simulink model "Assignment_2_RateAdaptive_UART"  (R2020a)
settings: Solver=FixedStepAuto  StartTime=0.0  StopTime=10.0  FixedStep=1e-3  RelTol=1e-3  EnableMultiTasking=on
undefined symbols (not defined in the file): A0, A1, D0, D1, D10, D11, D12, D13, D2, D3, D4, D5, D6, D7, D8, D9, PTA0, PTA1, PTA2, PTB2, PTB23, PTB3, PTB9, PTC16, PTC17, PTC2, PTC3, PTC4, PTD0, PTD1, PTD2, PTD3
libraries: frdmk64flib x22, etargetslib x5, dspstat3 x1, simulink x1
settings Model: ExtModeTrigDuration=5  Creator=School  LastModifiedBy=riley
settings OptimizationCC: EnhancedBackFolding=on  PassReuseOutputArgsAs=Individual arguments  ZeroExternalMemoryAtStartup=off  ZeroInternalMemoryAtStartup=off  MaxStackSize=64  OptimizeBlockOrder=speed  DifferentSizesBufferReuse=on  OptimizationCustomize=off  EfficientTunableParamExpr=on
settings DebuggingCC: ParameterTunabilityLossMsg=error
settings HardwareCC: ProdBitPerPointer=32  ProdBitPerSizeT=32  ProdBitPerPtrDiffT=32  ProdLargestAtomicInteger=Long  ProdLargestAtomicFloat=Double  ProdWordSize=32  ProdHWDeviceType=ARM Compatible->ARM Cortex
settings SFSimCC: MATLABDynamicMemAlloc=off
settings RTWCC: SystemTargetFile=ert.tlc  HardwareBoard=NXP FRDM-K64F  TemplateMakefile=ert_default_tmf  Toolchain=GNU Tools for ARM Embedded Processors
settings CodeAppCC: ForceParamTrailComments=on  IgnoreCustomStorageClasses=off  OperatorAnnotations=on  SimulinkDataObjDesc=on  SFDataObjDesc=on  InsertBlockDesc=on

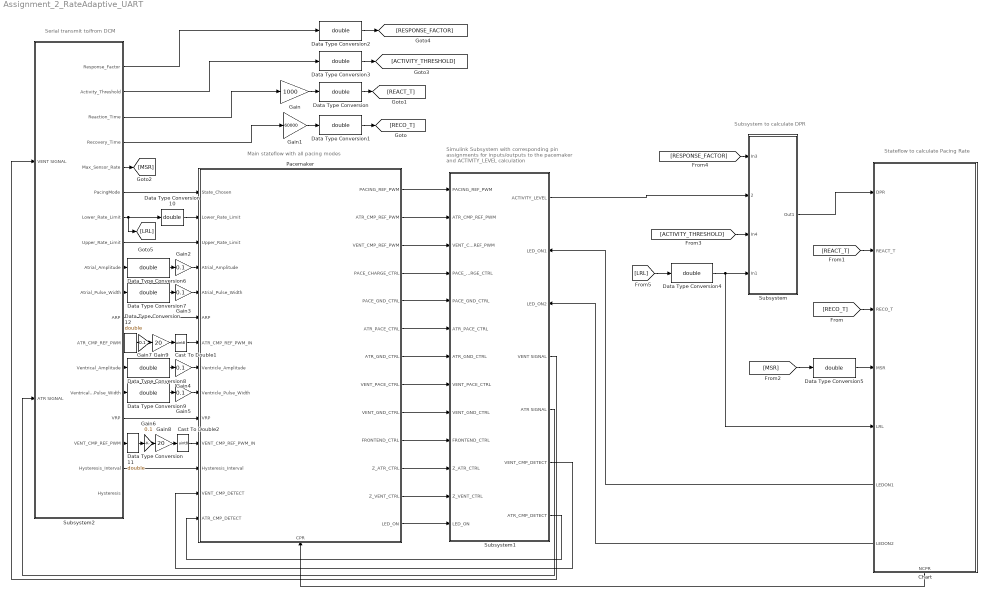
== system Assignment_2_RateAdaptive_UART ==
  note: Main stateflow with all pacing modes
  note: Serial transmit to/from DCM
  note: Stateflow to calculate Pacing Rate
  note: Subsystem to calculate DPR
  note: Simulink Subsystem with corresponding pin
      | assignments for inputs/outputs to the pacemaker
      | and ACTIVITY_LEVEL calculation
  Cast To Double1 : DataTypeConversion  OutDataTypeStr=uint8
  Cast To Double2 : DataTypeConversion  OutDataTypeStr=uint8
  Chart : Stateflow chart  TreatAsAtomicUnit=on
      settings: PortSchema="{\"entries\":[{\"content\":{\"sides\":[{\"content\":{\"connectorIds\":[\"In5\",\"In1\",\"In2\",\"In3\",\"In4\",\"Out2\",\"Out3\"]},\"type\":\"ConnectorPlacement.EquallySpacedRectSide\",\"uuid\":\"cb49ebd1-b2c7-4a1e-b062-18a1bf51e97f\"},{\"content\":{\"connectorIds\":[],\"side\":\"RIGHT\"},\"type\":\"ConnectorPlacement.EquallySpacedRectSide\",\"uuid\":\"35cf40a1-f02a-4965-9a15-2487395dd71b\"},{\"content\":{\"connectorIds\":[],\"side\":\"TOP\"},\"type\":\"ConnectorPlacement.EquallySpacedRectSide\",\"uuid\":\"8cf7664f-bebd-444c-a693-a1ee33fcaf3f\"},{\"content\":{\"connectorIds\":[\"Out1\"],\"side\":\"BOTTOM\"},\"type\":\"ConnectorPlacement.EquallySpacedRectSide\",\"uuid\":\"96b9c03b-a83e-462b-a12d-192e0bec7514\"}]},\"type\":\"ConnectorPlacement.EquallySpacedConnector\",\"uuid\":\"1030b27a-8fcd-482c-adda-aee1bfc69e16\"}],\"packageUris\":[\"http://schema.mathworks.com/mf0/Connector/19700101\"],\"version\":\"1.0\"}"
  Data Type Conversion{,1..12} (13 alike) : DataTypeConversion  OutDataTypeStr=double
  Gain : Gain  Gain=1000
  Gain1 : Gain  Gain=60000
  Gain{2..7} (6 alike) : Gain  Gain=0.1
  Gain8 : Gain  Gain=20
  Gain9 : Gain  Gain=20
  Pacemaker : Stateflow chart  TreatAsAtomicUnit=on
      settings: PortSchema="{\"entries\":[{\"content\":{\"sides\":[{\"content\":{\"connectorIds\":[\"In1\",\"In2\",\"In4\",\"In11\",\"In3\",\"In10\",\"In12\",\"In14\",\"In6\",\"In9\",\"In13\",\"In8\",\"In7\",\"In5\"]},\"type\":\"ConnectorPlacement.EquallySpacedRectSide\",\"uuid\":\"df877ca0-8245-4163-8fee-7182eab1d55d\"},{\"content\":{\"connectorIds\":[\"Out11\",\"Out12\",\"Out13\",\"Out2\",\"Out3\",\"Out1\",\"Out5\",\"Out7\",\"Out8\",\"Out10\",\"Out4\",\"Out9\",\"Out6\"],\"side\":\"RIGHT\"},\"type\":\"ConnectorPlacement.EquallySpacedRectSide\",\"uuid\":\"3a694184-6a85-4729-834f-a3ab7480664d\"},{\"content\":{\"connectorIds\":[],\"side\":\"TOP\"},\"type\":\"ConnectorPlacement.EquallySpacedRectSide\",\"uuid\":\"45b3d390-d3d3-4e22-8b52-b1590054c23a\"},{\"content\":{\"connectorIds\":[\"In15\"],\"side\":\"BOTTOM\"},\"type\":\"ConnectorPlacement.EquallySpacedRectSide\",\"uuid\":\"6c9e5202-d251-45f4-8fc3-f7acec5b4ccb\"}]},\"type\":\"ConnectorPlacement.EquallySpacedConnector\",\"uuid\":\"ad3b7ed4-c882-4247-8e15-d6beb1b6e9a6\"}],\"packageUris\":[\"http://schema.mathworks.com/mf0/Connector/19700101\"],\"version\":\"1.0\"}"
  Subsystem : Subsystem
  Subsystem1 : Subsystem
      settings: PortSchema="{\"entries\":[{\"content\":{\"sides\":[{\"content\":{\"connectorIds\":[\"In1\",\"In2\",\"In3\",\"In4\",\"In5\",\"In6\",\"In7\",\"In8\",\"In9\",\"In10\",\"In11\",\"In12\",\"In13\"]},\"type\":\"ConnectorPlacement.EquallySpacedRectSide\",\"uuid\":\"ef2db809-6ccb-4e10-b58a-4485458e2964\"},{\"content\":{\"connectorIds\":[\"Out1\",\"In14\",\"In15\",\"Out2\",\"Out3\",\"Out4\",\"Out5\"],\"side\":\"RIGHT\"},\"type\":\"ConnectorPlacement.EquallySpacedRectSide\",\"uuid\":\"23d27200-782c-4f65-a16b-b3dd9656ca92\"},{\"content\":{\"connectorIds\":[],\"side\":\"TOP\"},\"type\":\"ConnectorPlacement.EquallySpacedRectSide\",\"uuid\":\"4b957b3e-d3aa-4134-aa93-5dbe3bbb3ed9\"},{\"content\":{\"connectorIds\":[],\"side\":\"BOTTOM\"},\"type\":\"ConnectorPlacement.EquallySpacedRectSide\",\"uuid\":\"a8c808a9-b56b-4501-9a7a-854e8bc467f3\"}]},\"type\":\"ConnectorPlacement.EquallySpacedConnector\",\"uuid\":\"df464ebb-01b6-42d4-a9ed-9d5a529b4182\"}],\"packageUris\":[\"http://schema.mathworks.com/mf0/Connector/19700101\"],\"version\":\"1.0\"}"
  Subsystem2 : Subsystem
  wires:
  Pacemaker/2(PACE_CHARGE_CTRL) -> Subsystem1/4(PACE_CHARGE_CTRL)
  Chart/1(NCPR) -> Pacemaker/15(CPR)
  Chart/2(LEDON1) -> Subsystem1/14(LED_ON1)
  Pacemaker/7(VENT_PACE_CTRL) -> Subsystem1/8(VENT_PACE_CTRL)
  Chart/3(LEDON2) -> Subsystem1/15(LED_ON2)
  Pacemaker/6(LED_ON) -> Subsystem1/13(LED_ON)
  Pacemaker/9(Z_VENT_CTRL) -> Subsystem1/12(Z_VENT_CTRL)
  Pacemaker/10(FRONTEND_CTRL) -> Subsystem1/10(FRONTEND_CTRL)
  Pacemaker/12(ATR_CMP_REF_PWM) -> Subsystem1/2(ATR_CMP_REF_PWM)
  Pacemaker/11(PACING_REF_PWM) -> Subsystem1/1(PACING_REF_PWM)
  Pacemaker/13(VENT_CMP_REF_PWM) -> Subsystem1/3(VENT_CMP_REF_PWM)
  Pacemaker/5(ATR_GND_CTRL) -> Subsystem1/7(ATR_GND_CTRL)
  Pacemaker/1(ATR_PACE_CTRL) -> Subsystem1/6(ATR_PACE_CTRL)
  Pacemaker/8(VENT_GND_CTRL) -> Subsystem1/9(VENT_GND_CTRL)
  Subsystem/1(Out1) -> Chart/5(DPR)
  Pacemaker/3(PACE_GND_CTRL) -> Subsystem1/5(PACE_GND_CTRL)
  Subsystem1/4(" VENT_CMP_DETECT") -> Pacemaker/7(VENT_CMP_DETECT)
  Pacemaker/4(Z_ATR_CTRL) -> Subsystem1/11(Z_ATR_CTRL)
  Subsystem1/5(ATR_CMP_DETECT) -> Pacemaker/5(ATR_CMP_DETECT)
  [RESPONSE_FACTOR] -> Subsystem/1(In3)
  Subsystem1/1(ACTIVITY_LEVEL) -> Subsystem/2(2)
  Subsystem1/2(VENT SIGNAL) -> Subsystem2/1(VENT SIGNAL)
  Subsystem1/3(ATR SIGNAL) -> Subsystem2/2(ATR SIGNAL)
  Subsystem2/17(Hysteresis_Interval) -> Pacemaker/8(Hysteresis_Interval)
  Subsystem2/15(VRP) -> Pacemaker/9(VRP)
  Subsystem2/11(ARP) -> Pacemaker/10(ARP)
  Subsystem2/8(Upper_Rate_Limit) -> Pacemaker/4(Upper_Rate_Limit)
  Subsystem2/7(Lower_Rate_Limit) -> [LRL], Data Type Conversion10/1
  Subsystem2/6(PacingMode) -> Pacemaker/1(State_Chosen)
  Subsystem2/4(Recovery_Time) -> Gain1/1
  [RECO_T] -> Chart/2(RECO_T)
  Subsystem2/3(Reaction_Time) -> Gain/1
  [REACT_T] -> Chart/1(REACT_T)
  Subsystem2/5(Max_Sensor_Rate) -> [MSR]
  [ACTIVITY_THRESHOLD] -> Subsystem/3(In4)
  Gain/1 -> Data Type Conversion/1
  Data Type Conversion/1 -> [REACT_T]
  Data Type Conversion1/1 -> [RECO_T]
  Gain1/1 -> Data Type Conversion1/1
  Subsystem2/2(Activity_Threshold) -> Data Type Conversion3/1
  Subsystem2/1(Response_Factor) -> Data Type Conversion2/1
  Data Type Conversion2/1 -> [RESPONSE_FACTOR]
  Data Type Conversion3/1 -> [ACTIVITY_THRESHOLD]
  [LRL] -> Data Type Conversion4/1
  Data Type Conversion4/1 -> Chart/4(LRL), Subsystem/4(In1)
  [MSR] -> Data Type Conversion5/1
  Data Type Conversion5/1 -> Chart/3(MSR)
  Gain2/1 -> Pacemaker/11(Atrial_Amplitude)
  Subsystem2/9(Atrial_Amplitude) -> Data Type Conversion6/1
  Data Type Conversion6/1 -> Gain2/1
  Subsystem2/10(Atrial_Pulse_Width) -> Data Type Conversion7/1
  Gain3/1 -> Pacemaker/3(Atrial_Pulse_Width)
  Data Type Conversion7/1 -> Gain3/1
  Subsystem2/13(Ventrical_Amplitude) -> Data Type Conversion8/1
  Gain4/1 -> Pacemaker/14(Ventricle_Amplitude)
  Data Type Conversion8/1 -> Gain4/1
  Subsystem2/14(Ventrical_Pulse_Width) -> Data Type Conversion9/1
  Gain5/1 -> Pacemaker/6(Ventricle_Pulse_Width)
  Data Type Conversion9/1 -> Gain5/1
  Data Type Conversion10/1 -> Pacemaker/2(Lower_Rate_Limit)
  Subsystem2/16(VENT_CMP_REF_PWM) -> Data Type Conversion11/1
  Data Type Conversion11/1 -> Gain6/1
  Gain6/1 -> Gain8/1
  Gain8/1 -> Cast To Double2/1
  Cast To Double2/1 -> Pacemaker/13(VENT_CMP_REF_PWM_IN)
  Data Type Conversion12/1 -> Gain7/1
  Gain9/1 -> Cast To Double1/1
  Subsystem2/12(ATR_CMP_REF_PWM) -> Data Type Conversion12/1
  Gain7/1 -> Gain9/1
  Cast To Double1/1 -> Pacemaker/12(ATR_CMP_REF_PWM_IN)

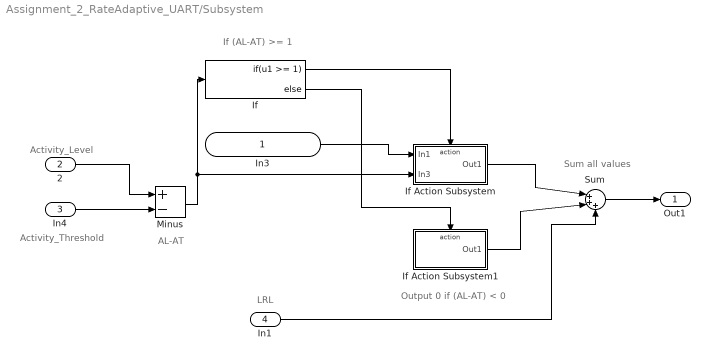
== system Assignment_2_RateAdaptive_UART/Subsystem ==
  note: Sum all values
  note: Output 0 if (AL-AT) < 0
  note: LRL
  note: AL-AT
  note: Activity_Threshold
  note: Activity_Level
  note: If (AL-AT) >= 1
  In3 : Inport
  2 : Inport  Port=2
  In4 : Inport  Port=3
  In1 : Inport  Port=4
  If : If  IfExpression=u1 >= 1
  If Action Subsystem : Subsystem  TreatAsAtomicUnit=on
  If Action Subsystem1 : Subsystem  TreatAsAtomicUnit=on
  Minus : Sum  Inputs=+-
  Sum : Sum  Inputs=|+++
  Out1 : Outport
  wires:
  2/1 -> Minus/1
  In4/1 -> Minus/2
  Minus/1 -> If Action Subsystem/2(In3), If/1
  If/1 -> If Action Subsystem/Action
  If/2 -> If Action Subsystem1/Action
  In3/1 -> If Action Subsystem/1(In1)
  Sum/1 -> Out1/1
  In1/1 -> Sum/3
  If Action Subsystem1/1(Out1) -> Sum/2
  If Action Subsystem/1(Out1) -> Sum/1

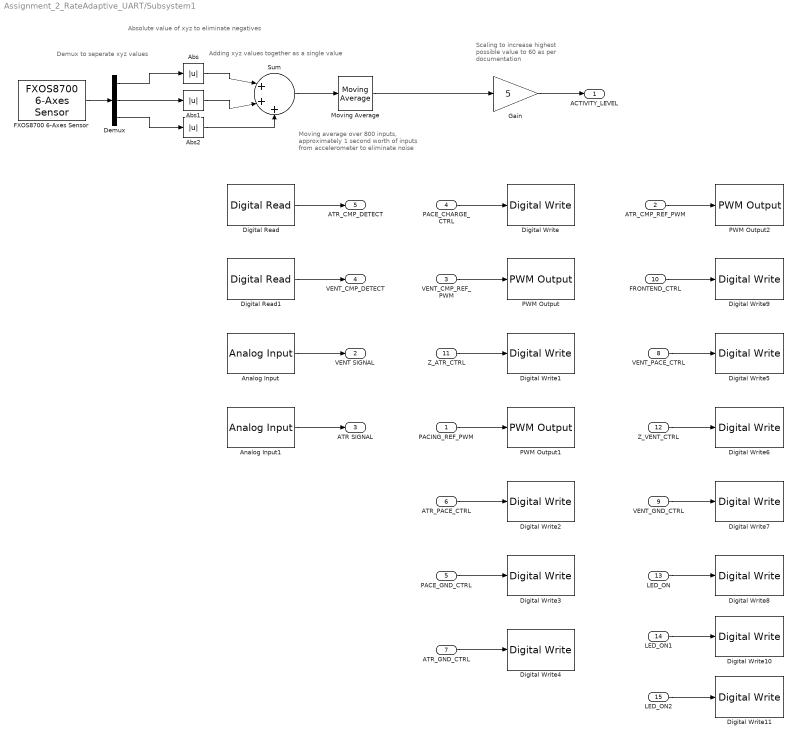
== system Assignment_2_RateAdaptive_UART/Subsystem1 ==
  note: Scaling to increase highest
      | possible value to 60
      | as per documentation
  note: Moving average over 800 inputs,
      | approximately 1 second worth of
      | inputs from accelerometer to eliminate
      | noise
  note: Adding xyz values together as a single value
  note: Absolute value of xyz to eliminate negatives
  note: Demux to seperate xyz values
  PACING_REF_PWM : Inport
  ATR_CMP_REF_PWM : Inport  Port=2
  VENT_CMP_REF_PWM : Inport  Port=3
  PACE_CHARGE_CTRL : Inport  Port=4
  PACE_GND_CTRL : Inport  Port=5
  ATR_PACE_CTRL : Inport  Port=6
  ATR_GND_CTRL : Inport  Port=7
  VENT_PACE_CTRL : Inport  Port=8
  VENT_GND_CTRL : Inport  Port=9
  FRONTEND_CTRL : Inport  Port=10
  Z_ATR_CTRL : Inport  Port=11
  Z_VENT_CTRL : Inport  Port=12
  LED_ON : Inport  Port=13
  LED_ON1 : Inport  Port=14
  LED_ON2 : Inport  Port=15
  Abs : Abs
  Abs1 : Abs
  Abs2 : Abs
  Analog Input : frdmk64flib/Analog Input  Whichpin=PTB3 (A1)  SampleTime=-1
  Analog Input1 : frdmk64flib/Analog Input  Whichpin=PTB2 (A0)  SampleTime=-1
  Demux : Demux  Outputs=3
  Digital Read : frdmk64flib/Digital Read  Whichpin=PTC16 (D0)  SampleTime=-1
  Digital Read1 : frdmk64flib/Digital Read  Whichpin=PTC17 (D1)  SampleTime=-1
  Digital Write : frdmk64flib/Digital Write  Whichpin=PTB9 (D2)
  Digital Write1 : frdmk64flib/Digital Write  Whichpin=PTB23 (D4)
  Digital Write10 : frdmk64flib/Digital Write  Whichpin=GREEN_LED
  Digital Write11 : frdmk64flib/Digital Write  Whichpin=BLUE_LED
  Digital Write2 : frdmk64flib/Digital Write  Whichpin=PTA0 (D8)
  Digital Write3 : frdmk64flib/Digital Write  Whichpin=PTD0 (D10)
  Digital Write4 : frdmk64flib/Digital Write  Whichpin=PTD2 (D11)
  Digital Write5 : frdmk64flib/Digital Write  Whichpin=PTC4 (D9)
  Digital Write6 : frdmk64flib/Digital Write  Whichpin=PTC3 (D7)
  Digital Write7 : frdmk64flib/Digital Write  Whichpin=PTD3 (D12)
  Digital Write8 : frdmk64flib/Digital Write  Whichpin=RED_LED
  Digital Write9 : frdmk64flib/Digital Write  Whichpin=PTD1 (D13)
  FXOS8700 6-Axes Sensor : frdmk64flib/FXOS8700 6-Axes Sensor  Activesensor=Accelerometer only  ODR=800Hz  HybridODR=400Hz  Accelfullrange=-4g to +4g  SampleTime=-1
  Gain : Gain  Gain=5
  Moving Average : dspstat3/Moving Average  Method=Sliding window  ForgettingFactorPort=off  SpecifyWindowLength=on  WindowLength=800  ForgettingFactor=0.9  SimulateUsing=Code generation
  PWM Output : frdmk64flib/PWM Output  Whichpin=PTA1 (D3)  InitialFrequency=2000  InitialDutyCycle=100
  PWM Output1 : frdmk64flib/PWM Output  Whichpin=PTA2 (D5)  InitialFrequency=2000  InitialDutyCycle=50
  PWM Output2 : frdmk64flib/PWM Output  Whichpin=PTC2 (D6)  InitialFrequency=2000  InitialDutyCycle=100
  Sum : Sum  Inputs=|+++
  ACTIVITY_LEVEL : Outport
  VENT SIGNAL : Outport  Port=2  OutDataTypeStr=double
  ATR SIGNAL : Outport  Port=3  OutDataTypeStr=double
  " VENT_CMP_DETECT" : Outport  Port=4
  ATR_CMP_DETECT : Outport  Port=5
  wires:
  Digital Read/1 -> ATR_CMP_DETECT/1
  Digital Read1/1 -> " VENT_CMP_DETECT"/1
  PACE_CHARGE_CTRL/1 -> Digital Write/1
  VENT_CMP_REF_PWM/1 -> PWM Output/1
  Z_ATR_CTRL/1 -> Digital Write1/1
  PACING_REF_PWM/1 -> PWM Output1/1
  ATR_PACE_CTRL/1 -> Digital Write2/1
  PACE_GND_CTRL/1 -> Digital Write3/1
  ATR_GND_CTRL/1 -> Digital Write4/1
  VENT_PACE_CTRL/1 -> Digital Write5/1
  Z_VENT_CTRL/1 -> Digital Write6/1
  VENT_GND_CTRL/1 -> Digital Write7/1
  LED_ON/1 -> Digital Write8/1
  ATR_CMP_REF_PWM/1 -> PWM Output2/1
  FRONTEND_CTRL/1 -> Digital Write9/1
  FXOS8700 6-Axes Sensor/1 -> Demux/1
  Demux/1 -> Abs/1
  Abs/1 -> Sum/1
  Abs1/1 -> Sum/2
  Demux/2 -> Abs1/1
  Demux/3 -> Abs2/1
  Abs2/1 -> Sum/3
  Gain/1 -> ACTIVITY_LEVEL/1
  Moving Average/1 -> Gain/1
  LED_ON1/1 -> Digital Write10/1
  LED_ON2/1 -> Digital Write11/1
  Sum/1 -> Moving Average/1
  Analog Input/1 -> VENT SIGNAL/1
  Analog Input1/1 -> ATR SIGNAL/1

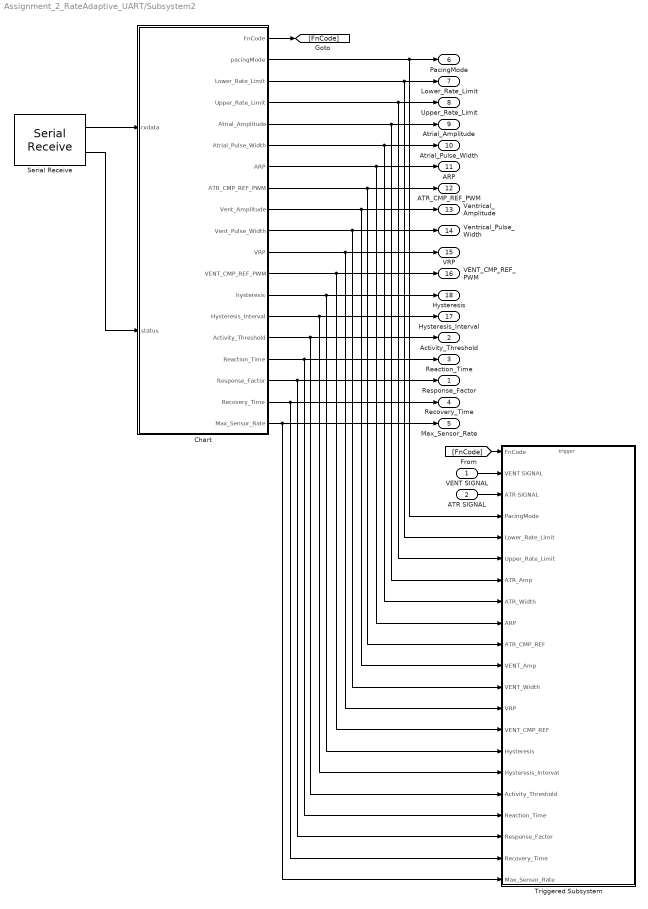
== system Assignment_2_RateAdaptive_UART/Subsystem2 ==
  VENT SIGNAL : Inport  OutDataTypeStr=double
  ATR SIGNAL : Inport  Port=2  OutDataTypeStr=double
  Chart : Stateflow chart  TreatAsAtomicUnit=on
      settings: PortSchema="{\"entries\":[{\"content\":{\"sides\":[{\"content\":{\"connectorIds\":[\"In1\",\"In2\"]},\"type\":\"ConnectorPlacement.EquallySpacedRectSide\",\"uuid\":\"c6a77858-5c94-45ee-95de-97b9ed53d3c1\"},{\"content\":{\"connectorIds\":[\"Out4\",\"Out2\",\"Out12\",\"Out17\",\"Out9\",\"Out10\",\"Out6\",\"Out7\",\"Out19\",\"Out5\",\"Out3\",\"Out18\",\"Out1\",\"Out11\",\"Out8\",\"Out14\",\"Out16\",\"Out15\",\"Out13\"],\"side\":\"RIGHT\"},\"type\":\"ConnectorPlacement.EquallySpacedRectSide\",\"uuid\":\"a361db13-9925-4434-9c10-dd06f36618c4\"},{\"content\":{\"connectorIds\":[],\"side\":\"TOP\"},\"type\":\"ConnectorPlacement.EquallySpacedRectSide\",\"uuid\":\"53233e8f-f176-4b90-8a25-5d32ffa06da9\"}]},\"type\":\"ConnectorPlacement.EquallySpacedConnector\",\"uuid\":\"c0e69ef7-0eb1-4c7e-8fb9-0ba3440918c3\"}],\"packageUris\":[\"http://schema.mathworks.com/mf0/Connector/19700101\"],\"version\":\"1.0\"}"
  Serial Receive : frdmk64flib/Serial Receive  SCIModule=0  Baudrate=uint32(9600)  Parity=None  StopBits=1  HardwareFlowControl=None  ByteOrder=LittleEndian  DataType=uint8  DataLength=23  BlockingMode=off  OutputStatus=on  SampleTime=-1
  Triggered Subsystem : Subsystem  TreatAsAtomicUnit=on
  Response_Factor : Outport
  Activity_Threshold : Outport  Port=2
  Reaction_Time : Outport  Port=3
  Recovery_Time : Outport  Port=4
  Max_Sensor_Rate : Outport  Port=5
  PacingMode : Outport  Port=6
  Lower_Rate_Limit : Outport  Port=7
  Upper_Rate_Limit : Outport  Port=8
  Atrial_Amplitude : Outport  Port=9
  Atrial_Pulse_Width : Outport  Port=10
  ARP : Outport  Port=11
  ATR_CMP_REF_PWM : Outport  Port=12
  Ventrical_Amplitude : Outport  Port=13
  Ventrical_Pulse_Width : Outport  Port=14
  VRP : Outport  Port=15
  VENT_CMP_REF_PWM : Outport  Port=16
  Hysteresis_Interval : Outport  Port=17
  Hysteresis : Outport  Port=18
  wires:
  Serial Receive/1 -> Chart/1(rxdata)
  Serial Receive/2 -> Chart/2(status)
  Chart/4(FnCode) -> [FnCode]
  Chart/2(pacingMode) -> Triggered Subsystem/4(PacingMode), PacingMode/1
  Chart/10(Atrial_Pulse_Width) -> Triggered Subsystem/8(ATR_Width), Atrial_Pulse_Width/1
  Chart/5(Vent_Pulse_Width) -> Triggered Subsystem/12(VENT_Width), Ventrical_Pulse_Width/1
  Chart/11(Hysteresis_Interval) -> Triggered Subsystem/16(Hysteresis_Interval), Hysteresis_Interval/1
  Chart/12(Lower_Rate_Limit) -> Triggered Subsystem/5(Lower_Rate_Limit), Lower_Rate_Limit/1
  Chart/9(Atrial_Amplitude) -> Triggered Subsystem/7(ATR_Amp), Atrial_Amplitude/1
  Chart/17(Upper_Rate_Limit) -> Triggered Subsystem/6(Upper_Rate_Limit), Upper_Rate_Limit/1
  Chart/6(ARP) -> Triggered Subsystem/9(ARP), ARP/1
  Chart/7(ATR_CMP_REF_PWM) -> Triggered Subsystem/10(ATR_CMP_REF), ATR_CMP_REF_PWM/1
  Chart/19(Vent_Amplitude) -> Triggered Subsystem/11(VENT_Amp), Ventrical_Amplitude/1
  Chart/3(VRP) -> Triggered Subsystem/13(VRP), VRP/1
  Chart/18(VENT_CMP_REF_PWM) -> Triggered Subsystem/14(VENT_CMP_REF), VENT_CMP_REF_PWM/1
  Chart/1(hysteresis) -> Triggered Subsystem/15(Hysteresis), Hysteresis/1
  Chart/8(Activity_Threshold) -> Triggered Subsystem/17(Activity_Threshold), Activity_Threshold/1
  Chart/14(Reaction_Time) -> Triggered Subsystem/18(Reaction_Time), Reaction_Time/1
  Chart/16(Response_Factor) -> Triggered Subsystem/19(Response_Factor), Response_Factor/1
  Chart/13(Max_Sensor_Rate) -> Triggered Subsystem/21(Max_Sensor_Rate), Max_Sensor_Rate/1
  Chart/15(Recovery_Time) -> Triggered Subsystem/20(Recovery_Time), Recovery_Time/1
  [FnCode] -> Triggered Subsystem/1(FnCode)
  VENT SIGNAL/1 -> Triggered Subsystem/2(VENT SIGNAL)
  ATR SIGNAL/1 -> Triggered Subsystem/3(ATR SIGNAL)

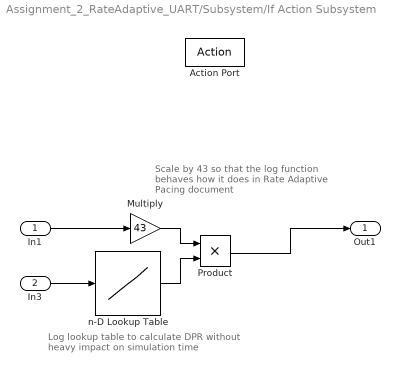
== system Assignment_2_RateAdaptive_UART/Subsystem/If Action Subsystem ==
  note: Scale by 43 so that the log function
      | behaves how it does in Rate
      | Adaptive Pacing document
  note: Log lookup table to calculate DPR
      | without heavy impact on simulation time
  In1 : Inport
  In3 : Inport  Port=2
  Action Port : ActionPort  ActionPortLabel=if(u1 >= 1)
  Multiply : Gain  Gain=43
  Product : Product  OutDataTypeStr=int8
  n-D Lookup Table : Lookup_n-D  NumberOfTableDimensions=1  LookupTableObject=log10  BreakpointsForDimension1=[1:55]  BreakpointsForDimension3=[5, 7]  Table="[0    0.3010    0.4771    0.6021    0.6990    0.7782    0.8451    0.9031    0.9542    1.0000    1.0414    1.0792    1.1139    1.1461    1.1761    1.2041    1.2304    1.2553    1.2788    1.3010    1.3222    1.3424    1.3617    1.3802    1.3979    1.4150    1.4314    1.4472    1.4624    1.4771    1.4914    1.5051    1.5185    1.5315    1.5441    1.5563    1.5682    1.5798    1.5911    1.6021    1.6128    1.6232    1.6335    1.6435    1.6532    1.6628    1.6721    1.6812    1.6902    1.6990    1.7076    1.7160    1.7243    1.7324    1.7404]"  InternalRulePriority=Speed  RndMeth=Simplest  InputSameDT=on
  Out1 : Outport
  wires:
  In1/1 -> Multiply/1
  In3/1 -> n-D Lookup Table/1
  Multiply/1 -> Product/1
  n-D Lookup Table/1 -> Product/2
  Product/1 -> Out1/1

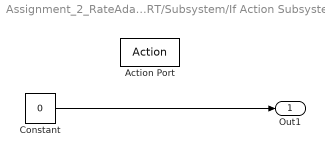
== system Assignment_2_RateAdaptive_UART/Subsystem/If Action Subsystem1 ==
  Action Port : ActionPort  ActionPortLabel=else
  Constant : Constant  Value=0
  Out1 : Outport
  wires:
  Constant/1 -> Out1/1

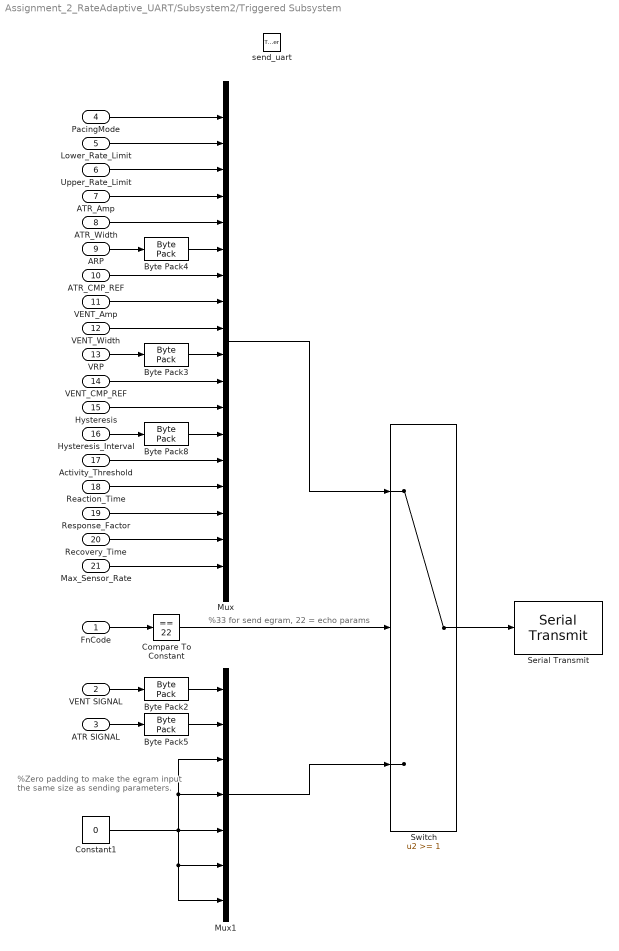
== system Assignment_2_RateAdaptive_UART/Subsystem2/Triggered Subsystem ==
  note: %Zero padding to make the egram input
      | the same size as sending parameters.
  note: %33 for send egram, 22 = echo params
  FnCode : Inport
  VENT SIGNAL : Inport  Port=2
  ATR SIGNAL : Inport  Port=3
  PacingMode : Inport  Port=4
  Lower_Rate_Limit : Inport  Port=5
  Upper_Rate_Limit : Inport  Port=6
  ATR_Amp : Inport  Port=7
  ATR_Width : Inport  Port=8
  ARP : Inport  Port=9
  ATR_CMP_REF : Inport  Port=10
  VENT_Amp : Inport  Port=11
  VENT_Width : Inport  Port=12
  VRP : Inport  Port=13
  VENT_CMP_REF : Inport  Port=14
  Hysteresis : Inport  Port=15
  Hysteresis_Interval : Inport  Port=16
  Activity_Threshold : Inport  Port=17
  Reaction_Time : Inport  Port=18
  Response_Factor : Inport  Port=19
  Recovery_Time : Inport  Port=20
  Max_Sensor_Rate : Inport  Port=21
  send_uart : TriggerPort  TriggerType=function-call  IsSimulinkFunction=on  FunctionName=send_uart  VariantControl=Variant  StatesWhenEnabling=reset
  Byte Pack2 : etargetslib/Byte Pack  datatypes={'double'}  byteAlign=1
  Byte Pack3 : etargetslib/Byte Pack  datatypes={'uint16'}  byteAlign=1
  Byte Pack4 : etargetslib/Byte Pack  datatypes={'uint16'}  byteAlign=1
  Byte Pack5 : etargetslib/Byte Pack  datatypes={'double'}  byteAlign=1
  Byte Pack8 : etargetslib/Byte Pack  datatypes={'uint16'}  byteAlign=1
  Compare To Constant : simulink/Logic and Bit Operations/Compare To Constant  relop===  const=22  OutDataTypeStr=boolean
  Constant1 : Constant  Value=0  OutDataTypeStr=uint8
  Mux : Mux  Inputs=18
  Mux1 : Mux  Inputs=7
  Serial Transmit : frdmk64flib/Serial Transmit  SCIModule=0  Baudrate=uint32(9600)  Parity=None  StopBits=1  HardwareFlowControl=None  ByteOrder=LittleEndian  BlockingMode=on  OutputStatus=off
  Switch : Switch  Threshold=1
  wires:
  Compare To Constant/1 -> Switch/2
  FnCode/1 -> Compare To Constant/1
  Hysteresis_Interval/1 -> Byte Pack8/1
  ARP/1 -> Byte Pack4/1
  VRP/1 -> Byte Pack3/1
  PacingMode/1 -> Mux/1
  Lower_Rate_Limit/1 -> Mux/2
  Upper_Rate_Limit/1 -> Mux/3
  Byte Pack4/1 -> Mux/6
  ATR_CMP_REF/1 -> Mux/7
  Byte Pack3/1 -> Mux/10
  VENT_CMP_REF/1 -> Mux/11
  Hysteresis/1 -> Mux/12
  Byte Pack8/1 -> Mux/13
  Activity_Threshold/1 -> Mux/14
  Reaction_Time/1 -> Mux/15
  Response_Factor/1 -> Mux/16
  Recovery_Time/1 -> Mux/17
  Max_Sensor_Rate/1 -> Mux/18
  Byte Pack2/1 -> Mux1/1
  VENT SIGNAL/1 -> Byte Pack2/1
  ATR SIGNAL/1 -> Byte Pack5/1
  Byte Pack5/1 -> Mux1/2
  Switch/1 -> Serial Transmit/1
  Mux1/1 -> Switch/3
  Mux/1 -> Switch/1
  ATR_Amp/1 -> Mux/4
  ATR_Width/1 -> Mux/5
  VENT_Amp/1 -> Mux/8
  VENT_Width/1 -> Mux/9
  Constant1/1 -> Mux1/5, Mux1/4, Mux1/3, Mux1/7, Mux1/6

== stateflow chart Assignment_2_RateAdaptive_UART/Pacemaker ==
  settings: executeAtInitialization=1
  state AOO
    state ChargingDischarging
      entry:
      %No Sensing
      FRONTEND_CTRL = false;
      %Charging
      PACE_CHARGE_CTRL = true;
      ATR_PACE_CTRL = false;
      VENT_PACE_CTRL = false;
      PACING_REF_PWM = (Atrial_Amplitude/5) * 100;
      %Discharging
      PACE_GND_CTRL = true;
      ATR_PACE_CTRL = false;
      ATR_GND_CTRL = true;
      VENT_PACE_CTRL = false;
      VENT_GND_CTRL = false;
      Z_ATR_CTRL = false;
      Z_VENT_CTRL = false;
      LED_ON = false;
      LRL = double(30000/Lower_Rate_Limit);
    state APacing
      entry:
      %Pace Atrial
      PACE_CHARGE_CTRL = false;
      PACE_GND_CTRL = true;
      ATR_PACE_CTRL = true;
      ATR_GND_CTRL = false;
      VENT_PACE_CTRL = false;
      VENT_GND_CTRL = false;
      Z_ATR_CTRL = false;
      Z_VENT_CTRL = false;
      LED_ON = true;
    note: % Charges until after the lower rate limit passes, sends a pulse for as long as the pulse width. Cycle repeats.
    note: % 30000 converted to msec better than 60000
        | when accelerometer connected.
    (default) -> AOO.ChargingDischarging
    AOO.ChargingDischarging -> AOO.APacing [order 1] : [after(LRL - Atrial_Pulse_Width, msec)]
    AOO.APacing -> AOO.ChargingDischarging : [after(Atrial_Pulse_Width,msec)]
  state VOO
    state ChargingDischarging
      entry:
      %No Sensing
      FRONTEND_CTRL = false;
      %Charging
      PACE_CHARGE_CTRL = true;
      ATR_PACE_CTRL = false;
      VENT_PACE_CTRL = false;
      PACING_REF_PWM = (Ventricle_Amplitude/5) * 100;
      %Discharging
      PACE_GND_CTRL = true;
      ATR_PACE_CTRL = false;
      ATR_GND_CTRL = false;
      VENT_PACE_CTRL = false;
      VENT_GND_CTRL = true;
      Z_ATR_CTRL = false;
      Z_VENT_CTRL = false;
      LED_ON = false;
      LRL = double(30000/Lower_Rate_Limit);
    state VPacing
      entry:
      %Pace Ventricle
      PACE_CHARGE_CTRL = false;
      PACE_GND_CTRL = true;
      ATR_PACE_CTRL = false;
      ATR_GND_CTRL = false;
      VENT_PACE_CTRL = true;
      VENT_GND_CTRL = false;
      Z_ATR_CTRL = false;
      Z_VENT_CTRL = false;
      LED_ON = true;
    note: % 30000 converted to msec better than 60000
        | when accelerometer connected.
    (default) -> VOO.ChargingDischarging
    VOO.ChargingDischarging -> VOO.VPacing [order 1] : [after(LRL - Ventricle_Pulse_Width, msec)]
    VOO.VPacing -> VOO.ChargingDischarging : [after(Ventricle_Pulse_Width,msec)]
  state AAI
    state APacing
      entry:
      %Disable Sensing
      FRONTEND_CTRL = false;
      %Pace Atrial
      PACE_CHARGE_CTRL = false;
      PACE_GND_CTRL = true;
      ATR_PACE_CTRL = true;
      ATR_GND_CTRL = false;
      VENT_PACE_CTRL = false;
      VENT_GND_CTRL = false;
      Z_ATR_CTRL = false;
      Z_VENT_CTRL = false;
      LED_ON = true;
    state ChargingDischarging
      entry:
      %Enable Sensing
      FRONTEND_CTRL = true;
      ATR_CMP_REF_PWM = 90
      %Charging
      PACE_CHARGE_CTRL = true;
      ATR_PACE_CTRL = false;
      VENT_PACE_CTRL = false;
      PACING_REF_PWM = (Atrial_Amplitude/5) * 100;
      %Discharging
      PACE_GND_CTRL = true;
      ATR_PACE_CTRL = false;
      ATR_GND_CTRL = true;
      VENT_PACE_CTRL = false;
      VENT_GND_CTRL = false;
      Z_ATR_CTRL = false;
      Z_VENT_CTRL = false;
      LED_ON = false;
      LRL = double(30000/Lower_Rate_Limit);
    state Hysteresis
      entry:
      %Enable Sensing
      FRONTEND_CTRL = true;
      %Charging
      PACE_CHARGE_CTRL = true;
      ATR_PACE_CTRL = false;
      VENT_PACE_CTRL = false;
      %Discharging
      PACE_GND_CTRL = true;
      ATR_PACE_CTRL = false;
      ATR_GND_CTRL = true;
      VENT_PACE_CTRL = false;
      VENT_GND_CTRL = false;
      Z_ATR_CTRL = false;
      Z_VENT_CTRL = false;
      LED_ON = false;
    note: % 30000 converted to msec better than 60000
        | when accelerometer connected.
    note: % If a natural heart beat is detected,
        | enter the Hysteresis state until no
        | natural beat occurs for the lower rate
        | limit plus the hysteresis interval
    (default) -> AAI.ChargingDischarging
    AAI.ChargingDischarging -> AAI.APacing [order 1] : [after(LRL - Atrial_Pulse_Width, msec)]
    AAI.APacing -> AAI.ChargingDischarging : [after(Atrial_Pulse_Width,msec)]
    AAI.Hysteresis -> AAI.APacing [order 1] : [after(LRL + Hysteresis_Interval, msec)]
    AAI.ChargingDischarging -> AAI.Hysteresis [order 2] : [after(ARP, msec) && ATR_CMP_DETECT == true]
    AAI.Hysteresis -> AAI.Hysteresis [order 2] : [after(ARP, msec) && ATR_CMP_DETECT == true]
  state VVI
    state ChargingDischarging
      entry:
      %Enable Sensing
      FRONTEND_CTRL = true;
      VENT_CMP_REF_PWM = 90
      %Charging
      PACE_CHARGE_CTRL = true;
      ATR_PACE_CTRL = false;
      VENT_PACE_CTRL = false;
      PACING_REF_PWM = (Ventricle_Amplitude/5) * 100;
      %Discharging
      PACE_GND_CTRL = true;
      ATR_PACE_CTRL = false;
      ATR_GND_CTRL = false;
      VENT_PACE_CTRL = false;
      VENT_GND_CTRL = true;
      Z_ATR_CTRL = false;
      Z_VENT_CTRL = false;
      LED_ON = false;
      LRL = double(30000/Lower_Rate_Limit);
    state VPacing
      entry:
      %Disable Sensing
      FRONTEND_CTRL = false;
      %Pace Ventricle
      PACE_CHARGE_CTRL = false;
      PACE_GND_CTRL = true;
      ATR_PACE_CTRL = false;
      ATR_GND_CTRL = false;
      VENT_PACE_CTRL = true;
      VENT_GND_CTRL = false;
      Z_ATR_CTRL = false;
      Z_VENT_CTRL = false;
      LED_ON = true;
    state Hysteresis
      entry:
      %Enable Sensing
      FRONTEND_CTRL = true;
      %Charging
      PACE_CHARGE_CTRL = true;
      ATR_PACE_CTRL = false;
      VENT_PACE_CTRL = false;
      %Discharging
      PACE_GND_CTRL = true;
      ATR_PACE_CTRL = false;
      ATR_GND_CTRL = false;
      VENT_PACE_CTRL = false;
      VENT_GND_CTRL = true;
      Z_ATR_CTRL = false;
      Z_VENT_CTRL = false;
      LED_ON = false;
    note: % 30000 converted to msec better than 60000
        | when accelerometer connected.
    (default) -> VVI.ChargingDischarging
    VVI.ChargingDischarging -> VVI.VPacing [order 1] : [after(LRL - Ventricle_Pulse_Width, msec)]
    VVI.VPacing -> VVI.ChargingDischarging : [after(Ventricle_Pulse_Width,msec)]
    VVI.Hysteresis -> VVI.VPacing [order 2] : [after(LRL + Hysteresis_Interval, msec)]
    VVI.ChargingDischarging -> VVI.Hysteresis [order 2] : [after(VRP, msec) && VENT_CMP_DETECT==true]
    VVI.Hysteresis -> VVI.Hysteresis [order 1] : [after(VRP, msec) && VENT_CMP_DETECT==true]
  state initialState
  state IDLE
  note: % Upon startup, pacemaker goes into the selected
      | mode based on the "State_Chosen" variable. State
      | changes if new State_Chosen input is detected
  state AOOR
    state ChargingDischarging
      entry:
      %No Sensing
      FRONTEND_CTRL = false;
      %Charging
      PACE_CHARGE_CTRL = true;
      ATR_PACE_CTRL = false;
      VENT_PACE_CTRL = false;
      PACING_REF_PWM = (Atrial_Amplitude/5) * 100;
      %Discharging
      PACE_GND_CTRL = true;
      ATR_PACE_CTRL = false;
      ATR_GND_CTRL = true;
      VENT_PACE_CTRL = false;
      VENT_GND_CTRL = false;
      Z_ATR_CTRL = false;
      Z_VENT_CTRL = false;
      LED_ON = false;
      PACE = 30000/CPR;
    state APacing
      entry:
      %Pace Atrial
      PACE_CHARGE_CTRL = false;
      PACE_GND_CTRL = true;
      ATR_PACE_CTRL = true;
      ATR_GND_CTRL = false;
      VENT_PACE_CTRL = false;
      VENT_GND_CTRL = false;
      Z_ATR_CTRL = false;
      Z_VENT_CTRL = false;
      LED_ON = true;
    note: % Charges until after the lower rate limit passes, sends a pulse for as long as the pulse width. Cycle repeats.
    note: % 30000 converted to msec better than 60000
        | when accelerometer connected.
    (default) -> AOOR.ChargingDischarging
    AOOR.ChargingDischarging -> AOOR.APacing [order 1] : [after(PACE - Atrial_Pulse_Width, msec)]
    AOOR.APacing -> AOOR.ChargingDischarging : [after(Atrial_Pulse_Width,msec)]
  state VOOR
    state ChargingDischarging
      entry:
      %No Sensing
      FRONTEND_CTRL = false;
      %Charging
      PACE_CHARGE_CTRL = true;
      ATR_PACE_CTRL = false;
      VENT_PACE_CTRL = false;
      PACING_REF_PWM = (Ventricle_Amplitude/5) * 100;
      %Discharging
      PACE_GND_CTRL = true;
      ATR_PACE_CTRL = false;
      ATR_GND_CTRL = false;
      VENT_PACE_CTRL = false;
      VENT_GND_CTRL = true;
      Z_ATR_CTRL = false;
      Z_VENT_CTRL = false;
      LED_ON = false;
      PACE = 30000/CPR;
    state VPacing
      entry:
      %Pace Ventricle
      PACE_CHARGE_CTRL = false;
      PACE_GND_CTRL = true;
      ATR_PACE_CTRL = false;
      ATR_GND_CTRL = false;
      VENT_PACE_CTRL = true;
      VENT_GND_CTRL = false;
      Z_ATR_CTRL = false;
      Z_VENT_CTRL = false;
      LED_ON = true;
    note: % 30000 converted to msec better than 60000
        | when accelerometer connected.
    (default) -> VOOR.ChargingDischarging
    VOOR.ChargingDischarging -> VOOR.VPacing [order 1] : [after(PACE - Ventricle_Pulse_Width, msec)]
    VOOR.VPacing -> VOOR.ChargingDischarging : [after(Ventricle_Pulse_Width,msec)]
  state AAIR
    state APacing
      entry:
      %Disable Sensing
      FRONTEND_CTRL = false;
      %Pace Atrial
      PACE_CHARGE_CTRL = false;
      PACE_GND_CTRL = true;
      ATR_PACE_CTRL = true;
      ATR_GND_CTRL = false;
      VENT_PACE_CTRL = false;
      VENT_GND_CTRL = false;
      Z_ATR_CTRL = false;
      Z_VENT_CTRL = false;
      LED_ON = true;
    state ChargingDischarging
      entry:
      %Enable Sensing
      FRONTEND_CTRL = true;
      ATR_CMP_REF_PWM = ATR_CMP_REF_PWM_IN
      %Charging
      PACE_CHARGE_CTRL = true;
      ATR_PACE_CTRL = false;
      VENT_PACE_CTRL = false;
      PACING_REF_PWM = (Atrial_Amplitude/5) * 100;
      %Discharging
      PACE_GND_CTRL = true;
      ATR_PACE_CTRL = false;
      ATR_GND_CTRL = true;
      VENT_PACE_CTRL = false;
      VENT_GND_CTRL = false;
      Z_ATR_CTRL = false;
      Z_VENT_CTRL = false;
      LED_ON = false;
      PACE = 30000/CPR;
    state Hysteresis
      entry:
      %Enable Sensing
      FRONTEND_CTRL = true;
      %Charging
      PACE_CHARGE_CTRL = true;
      ATR_PACE_CTRL = false;
      VENT_PACE_CTRL = false;
      %Discharging
      PACE_GND_CTRL = true;
      ATR_PACE_CTRL = false;
      ATR_GND_CTRL = true;
      VENT_PACE_CTRL = false;
      VENT_GND_CTRL = false;
      Z_ATR_CTRL = false;
      Z_VENT_CTRL = false;
      LED_ON = false;
    note: % 30000 converted to msec better than 60000
        | when accelerometer connected.
    note: % If a natural heart beat is detected,
        | enter the Hysteresis state until no
        | natural beat occurs for the lower rate
        | limit plus the hysteresis interval
    (default) -> AAIR.ChargingDischarging
    AAIR.ChargingDischarging -> AAIR.APacing [order 1] : [after(PACE - Atrial_Pulse_Width, msec)]
    AAIR.APacing -> AAIR.ChargingDischarging : [after(Atrial_Pulse_Width,msec)]
    AAIR.Hysteresis -> AAIR.APacing [order 1] : [after(PACE + Hysteresis_Interval, msec)]
    AAIR.ChargingDischarging -> AAIR.Hysteresis [order 2] : [after(ARP, msec) && ATR_CMP_DETECT == true]
    AAIR.Hysteresis -> AAIR.Hysteresis [order 2] : [after(ARP, msec) && ATR_CMP_DETECT == true]
  state VVIR
    state ChargingDischarging
      entry:
      %Enable Sensing
      FRONTEND_CTRL = true;
      VENT_CMP_REF_PWM = VENT_CMP_REF_PWM_IN
      %Charging
      PACE_CHARGE_CTRL = true;
      ATR_PACE_CTRL = false;
      VENT_PACE_CTRL = false;
      PACING_REF_PWM = (Ventricle_Amplitude/5) * 100;
      %Discharging
      PACE_GND_CTRL = true;
      ATR_PACE_CTRL = false;
      ATR_GND_CTRL = false;
      VENT_PACE_CTRL = false;
      VENT_GND_CTRL = true;
      Z_ATR_CTRL = false;
      Z_VENT_CTRL = false;
      LED_ON = false;
      PACE = 30000/CPR;
    state VPacing
      entry:
      %Disable Sensing
      FRONTEND_CTRL = false;
      %Pace Ventricle
      PACE_CHARGE_CTRL = false;
      PACE_GND_CTRL = true;
      ATR_PACE_CTRL = false;
      ATR_GND_CTRL = false;
      VENT_PACE_CTRL = true;
      VENT_GND_CTRL = false;
      Z_ATR_CTRL = false;
      Z_VENT_CTRL = false;
      LED_ON = true;
    state Hysteresis
      entry:
      %Enable Sensing
      FRONTEND_CTRL = true;
      %Charging
      PACE_CHARGE_CTRL = true;
      ATR_PACE_CTRL = false;
      VENT_PACE_CTRL = false;
      %Discharging
      PACE_GND_CTRL = true;
      ATR_PACE_CTRL = false;
      ATR_GND_CTRL = false;
      VENT_PACE_CTRL = false;
      VENT_GND_CTRL = true;
      Z_ATR_CTRL = false;
      Z_VENT_CTRL = false;
      LED_ON = false;
    note: % 30000 converted to msec better than 60000
        | when accelerometer connected.
    (default) -> VVIR.ChargingDischarging
    VVIR.ChargingDischarging -> VVIR.VPacing [order 1] : [after(PACE - Ventricle_Pulse_Width, msec)]
    VVIR.VPacing -> VVIR.ChargingDischarging : [after(Ventricle_Pulse_Width,msec)]
    VVIR.Hysteresis -> VVIR.VPacing : [after(PACE + Hysteresis_Interval, msec)]
    VVIR.ChargingDischarging -> VVIR.Hysteresis [order 2] : [after(VRP, msec) && VENT_CMP_DETECT==true]
  VVI.ChargingDischarging -> initialState [order 3] : [State_Chosen~=4]
  AAI.ChargingDischarging -> initialState [order 3] : [State_Chosen~=3]
  VOOR.ChargingDischarging -> initialState [order 2] : [State_Chosen~=6]
  VVIR.ChargingDischarging -> initialState [order 3] : [State_Chosen~=8]
  AAIR.ChargingDischarging -> initialState [order 3] : [State_Chosen~=7]
  AOO.ChargingDischarging -> initialState [order 2] : [State_Chosen~=1]
  AOOR.ChargingDischarging -> initialState [order 2] : [State_Chosen~=5]
  VOO.ChargingDischarging -> initialState [order 2] : [State_Chosen~=2]
  initialState -> AOO [order 1] : [State_Chosen==1]
  initialState -> VOO [order 2] : [State_Chosen==2]
  initialState -> AAI [order 3] : [State_Chosen==3]
  initialState -> VVI [order 4] : [State_Chosen==4]
  (default) -> IDLE
  initialState -> IDLE [order 9] : [State_Chosen==0]
  IDLE -> initialState
  initialState -> AOOR [order 8] : [State_Chosen==5]
  initialState -> VOOR [order 5] : [State_Chosen==6]
  initialState -> AAIR [order 6] : [State_Chosen==7]
  initialState -> VVIR [order 7] : [State_Chosen==8]
  data: State_Chosen input uint8; Lower_Rate_Limit input double; Atrial_Pulse_Width input double; Upper_Rate_Limit input uint8; ATR_PACE_CTRL output boolean =false; PACE_CHARGE_CTRL output boolean =false; PACE_GND_CTRL output boolean =false; Z_ATR_CTRL output boolean =false; ATR_GND_CTRL output boolean =false; LED_ON output boolean; VENT_PACE_CTRL output boolean; VENT_GND_CTRL output; Z_VENT_CTRL output; ATR_CMP_DETECT input boolean; Ventricle_Pulse_Width input double; VENT_CMP_DETECT input boolean; Hysteresis_Interval input uint16; FRONTEND_CTRL output; VRP input uint16; ARP input uint16; PACING_REF_PWM output; ATR_CMP_REF_PWM output; VENT_CMP_REF_PWM output; Atrial_Amplitude input double; ATR_CMP_REF_PWM_IN input uint8; VENT_CMP_REF_PWM_IN input uint8; Ventricle_Amplitude input double; CPR input; LRL local double; PACE local

== stateflow chart Assignment_2_RateAdaptive_UART/Subsystem2/Chart ==
  settings: executeAtInitialization=1
  note: %When parameters are requested to be updated, don't send egram data.
  state SET_PARAM
    entry:
    FnCode = rxdata(2);
    pacingMode = rxdata(3);
    Lower_Rate_Limit = rxdata(4);
    Upper_Rate_Limit = rxdata(5);
    Atrial_Amplitude = rxdata(6);
    Atrial_Pulse_Width = rxdata(7);
    ARP = typecast(rxdata(8:9), 'uint16');
    ATR_CMP_REF_PWM = rxdata(10);
    Vent_Amplitude = rxdata(11);
    Vent_Pulse_Width = rxdata(12);
    VRP = typecast(rxdata(13:14), 'uint16');
    VENT_CMP_REF_PWM = rxdata(15)
    hysteresis = rxdata(16);
    Hysteresis_Interval = typecast(rxdata(17:18), 'uint16');
    Activity_Threshold = rxdata(19);
    Reaction_Time = rxdata(20);
    Response_Factor = rxdata(21);
    Recovery_Time = rxdata(22);
    Max_Sensor_Rate = rxdata(23);
  note: %Constantly send egram data when requested by the DCM
      | until another uart transmission is received
  state INITIAL
    entry:
    %Default nominal values
    FnCode = 22; %Echo params by default
    pacingMode = 0; %Start in IDLE for safety
    Lower_Rate_Limit = 60; % 60BPM
    Upper_Rate_Limit = 120;
    Atrial_Amplitude = 35; %decimal, /10
    Atrial_Pulse_Width = 4; %decimal, /10
    ARP = 250;
    ATR_CMP_REF_PWM = 45; %decimal, /10
    Vent_Amplitude = 35; %decimal, /10
    Vent_Pulse_Width = 04; %decimal, /10
    VRP = 320;
    VENT_CMP_REF_PWM = 45; %decimal, /10
    hysteresis = 0; %Set hysteresis to 0 if = 0
    Hysteresis_Interval = 300; % ms
    Activity_Threshold = 15;
    Reaction_Time = 10;
    Response_Factor = 8;
    Recovery_Time = 5; %Minutes
    Max_Sensor_Rate = 60;
  state STANDBY
    %If no valid FnCode is received
    %treat as stop code.
    %Stay in standby, do not send any data
  state SEND_EGRAM
    send_uart();
    FnCode = rxdata(2);
  state ECHO_PARAM
    entry:
    send_uart();
    FnCode = rxdata(2);
  SET_PARAM -> STANDBY
  (junction 13) -> SET_PARAM [order 1] : [rxdata(2) == 0x0b]
  (default) -> INITIAL
  (junction 8) -> STANDBY [order 2]
  SEND_EGRAM -> SEND_EGRAM [order 2]
  INITIAL -> STANDBY
  (junction 13) -> SEND_EGRAM [order 3] : [rxdata(2) == 0x21]
  (junction 8) -> (junction 13) [order 1] : [rxdata(1) == 0x10]
  STANDBY -> (junction 8) : [status == 0]
  (junction 13) -> ECHO_PARAM [order 2] : [rxdata(2) == 0x16]
  SEND_EGRAM -> (junction 8) [order 1] : [status == 0]
  ECHO_PARAM -> STANDBY
  data: rxdata input uint8; status input uint8; hysteresis output uint8; pacingMode output uint8; VRP output uint16; FnCode output uint8; Vent_Pulse_Width output uint8; ARP output uint16; ATR_CMP_REF_PWM output uint8; Activity_Threshold output uint8; Atrial_Amplitude output uint8; Atrial_Pulse_Width output uint8; Hysteresis_Interval output uint16; Lower_Rate_Limit output uint8; Max_Sensor_Rate output uint8; Reaction_Time output uint8; Recovery_Time output uint8; Response_Factor output uint8; Upper_Rate_Limit output uint8; VENT_CMP_REF_PWM output uint8; Vent_Amplitude output uint8

== stateflow chart Assignment_2_RateAdaptive_UART/Chart ==
  state State1
    entry:
    NCPR = LRL;
  note: Buffer to avoid potential wrong values from being
      | sent to stateflow from accelerometer
  state Increasing
    entry:
    ROC = (MSR-LRL)/REACT_T;
    if NCPR > MSR
    NCPR = MSR;
    elseif NCPR <= LRL
    NCPR = LRL;
    elseif NCPR >= DPR
    NCPR = DPR;
    end
    LEDON1 = true;
    LEDON2 = false;
  state Decreasing
    entry:
    ROC = (MSR-LRL)/RECO_T;
    if NCPR <= LRL
    NCPR = LRL;
    elseif NCPR > MSR
    NCPR = MSR;
    elseif NCPR <= DPR
    NCPR = DPR;
    end
    LEDON1 = false;
    LEDON2 = true;
  note: ROC brings NCPR up from LRL to MSR
      | over RECO_T. If statements restrict NCPR
      | to be between constraints (LRL, MSR, DPR)
  note: ROC brings NCPR down from MSR to LRL
      | over RECO_T. If statements restrict NCPR
      | to be between constraints (LRL, MSR, DPR)
  (default) -> State1
  State1 -> Decreasing : [after(10, msec)]
  Decreasing -> Increasing [order 1] : [DPR > NCPR]
  Decreasing -> Decreasing [order 2] : [after(1, msec)]{NCPR = NCPR - ROC}
  Increasing -> Increasing [order 2] : [after(1, msec)]{NCPR = NCPR + ROC}
  Increasing -> Decreasing [order 1] : [DPR < NCPR]
  data: REACT_T input double; RECO_T input double; MSR input double; LRL input double; NCPR output double; DPR input; LEDON1 output; LEDON2 output; ROC local
